simulink model "suma_senales"  (R2023b)
settings: Solver=VariableStepAuto  StartTime=0.0  StopTime=10.0  RelTol=1e-3
libraries: simulink x1
settings Model: Creator=20808  LastModifiedBy=20808

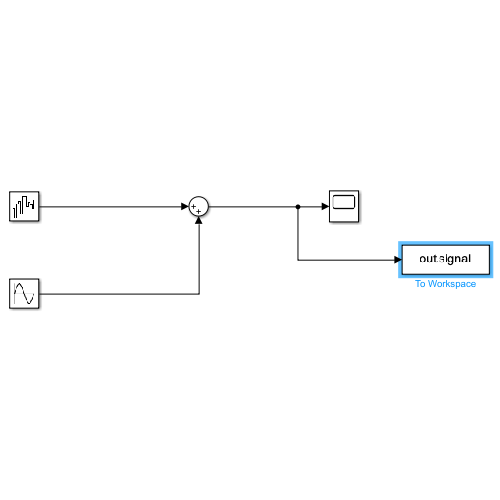
[thumbnail: Simulink's stored preview of the top-level diagram]
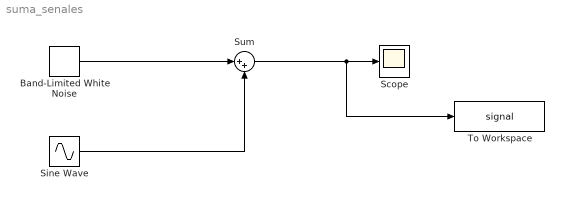
== system suma_senales ==
  Band-Limited White Noise : simulink/Sources/Band-Limited White Noise  Cov=[0.1]  Ts=0.1  seed=[23341]
  Scope : Scope
  Sine Wave : Sin  Amplitude=10  SampleTime=0
  Sum : Sum  Inputs=|++
  To Workspace : ToWorkspace  VariableName=signal  SampleTime=-1
  wires:
  Band-Limited White Noise/1 -> Sum/1
  Sine Wave/1 -> Sum/2
  Sum/1 -> To Workspace/1, Scope/1
